simulink model "six_rod_tensegrity_model_2021a"  (R2021a)
settings: Solver=ode45  StartTime=0  StopTime=Inf  RelTol=1e-1
values from neighbouring files (symbols this model uses):
  grivity_z = -9.80665    [code_for_6_rods_tensegrity.m]
  i = 19    [drive_params.m]
  Jsum = Jd + Jp + Jnagr    (= 9.27e-08)    [drive_params.m]
  km = 9.32 / 1000    (= 0.00932)    [drive_params.m]
  kpdr = 0.81    [drive_params.m]
  kw = 60 / (2*pi * 1020)    (= 0.00936205547599)    [drive_params.m]
  L = 0.14 / 1000    (= 0.00014)    [drive_params.m]
  load_mass = 0.5    [code_for_6_rods_tensegrity.m]
  plane_offset = -(rod_length/2 + 0.032 + rod_radius)    [code_for_6_rods_tensegrity.m]
  R = 5.3    [drive_params.m]
  rod_end_drive_offset = spool_active_length    (= 0.015)    [code_for_6_rods_tensegrity.m]
  rod_end_mass = 0.05    [code_for_6_rods_tensegrity.m]
  rod_end_mass_with_drive = 0.2    [code_for_6_rods_tensegrity.m]
  rod_mass = 0.028    [code_for_6_rods_tensegrity.m]
  rod_mass_with_drive = 0.038    [code_for_6_rods_tensegrity.m]
  rod_radius = 0.004    [code_for_6_rods_tensegrity.m]
undefined symbols (not defined in the file or in its folder): Left_end_cap_1_1, Left_end_cap_2_3, Left_end_cap_3_5, Left_end_cap_4_7, Left_end_cap_5_9, Left_end_cap_6_11, Right_end_cap_1_2, Right_end_cap_2_4, Right_end_cap_3_6, Right_end_cap_4_8, Right_end_cap_5_10, Right_end_cap_6_12, Rod_center_1, Rod_center_2, Rod_center_3, Rod_center_4, Rod_center_5, Rod_center_6, sigbuilder_block, X, Y, Z
libraries: sm_lib x403, nesl_utility x73
(part 2 of 5)

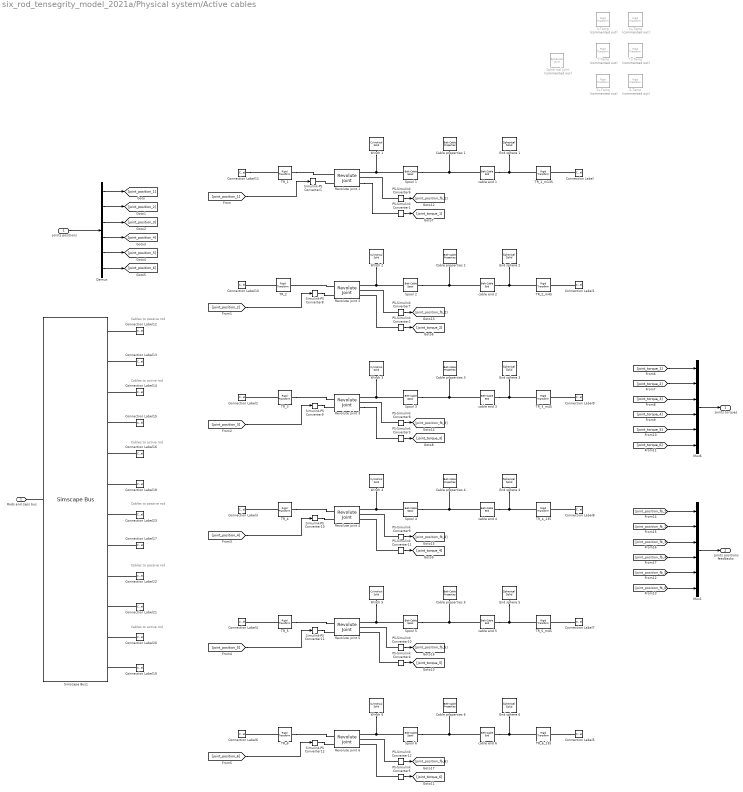
== system six_rod_tensegrity_model_2021a/Physical system/Active cables ==
  note: Cables to passive rod
  note: Cables to active rod
  note: Cables to active rod
  note: Cables to passive rod
  note: Cables to passive rod
  note: Cables to active rod
  Joints positions : Inport
  Cable properties {1..6} (6 alike) : sm_lib/Belts and Cables/Belt-Cable Properties  DrumBeltCableAlignment=Unrestricted  GraphicType=PitchLine  GraphicVisPropType=SimpleVisualProperties  GraphicDiffuseColor=cable_color  GraphicSpecularColor=[0.5 0.5 0.5 1.0]  GraphicAmbientColor=[0.15 0.15 0.15 1.0]  GraphicEmissiveColor=[0.0 0.0 0.0 1.0]  GraphicShininess=75  GraphicOpacity=1
      settings: SourceProductBaseCode=MS
  Connection Label : ConnectionLabel  Label=Cable_left_1_1
  Connection Label1 : ConnectionLabel  Label=Cable_left_2_2
  Connection Label10 : ConnectionLabel  Label=Cable_right_2_6
  Connection Label11 : ConnectionLabel  Label=Cable_right_1_12
  Connection Label12 : ConnectionLabel  Label=Cable_left_1_1
  Connection Label13 : ConnectionLabel  Label=Cable_left_2_2
  Connection Label14 : ConnectionLabel  Label=Cable_left_3_3
  Connection Label15 : ConnectionLabel  Label=Cable_left_4_4
  Connection Label16 : ConnectionLabel  Label=Cable_left_5_5
  Connection Label17 : ConnectionLabel  Label=Cable_left_6_8
  Connection Label18 : ConnectionLabel  Label=Cable_right_2_6
  Connection Label19 : ConnectionLabel  Label=Cable_right_1_12
  Connection Label2 : ConnectionLabel  Label=Cable_left_3_3
  Connection Label20 : ConnectionLabel  Label=Cable_right_6_11
  Connection Label21 : ConnectionLabel  Label=Cable_right_5_10
  Connection Label22 : ConnectionLabel  Label=Cable_right_4_9
  Connection Label23 : ConnectionLabel  Label=Cable_right_3_7
  Connection Label3 : ConnectionLabel  Label=Cable_left_4_4
  Connection Label4 : ConnectionLabel  Label=Cable_left_5_5
  Connection Label5 : ConnectionLabel  Label=Cable_left_6_8
  Connection Label6 : ConnectionLabel  Label=Cable_right_6_11
  Connection Label7 : ConnectionLabel  Label=Cable_right_5_10
  Connection Label8 : ConnectionLabel  Label=Cable_right_4_9
  Connection Label9 : ConnectionLabel  Label=Cable_right_3_7
  Demux : Demux  Outputs=6
  End sphere {1..6} (6 alike) : sm_lib/Body Elements/Spherical Solid  GraphicAmbientColor=[0.15 0.15 0.15 1.0]  BasedOnType=Density  CenterOfMass=[0 0 0]  CenterOfMassUnits=m  GraphicDiffuseColor=spool_color  Density=spool_active_density  DensityUnits=kg/m^3  DoExposeReferenceFrame=on  GraphicEmissiveColor=[0.0 0.0 0.0 1.0]  ExportEntireGeometry=off  SerializedExposedGeometries=<ExposedGeometries/>  SerializedFrames=<Frames/>  MarkerShape=Frame  MarkerSize=10  GraphicType=FromGeometry  InertiaType=CalculateFromGeometry  Mass=0.01  MassUnits=kg  MomentsOfInertia=[1 1 1]  MomentsOfInertiaUnits=kg*m^2  GraphicOpacity=1.0  ProductsOfInertia=[0 0 0]  ProductsOfInertiaUnits=kg*m^2  GraphicShininess=10  GraphicSpecularColor=[0.8 0.8 0.8]  SphereRadius=spool_active_end_radius  SphereRadiusUnits=m  GraphicVisPropType=SimpleVisualProperties
  Mux1 : Mux  Inputs=6
  Mux6 : Mux  Inputs=6
  PS-Simulink Converter{1..5,11} (6 alike) : nesl_utility/PS-Simulink Converter  PhysicalDomain=network_engine_domain  SubClassName=ps_output  LeftPortType=input  RightPortType=output  PseudoPeriodic=off  Frequencies=[]  Unit=N*m  AffineConversion=off
      settings: SourceProductBaseCode=PW,SS
  PS-Simulink Converter{6..10,12} (6 alike) : nesl_utility/PS-Simulink Converter  PhysicalDomain=network_engine_domain  SubClassName=ps_output  LeftPortType=input  RightPortType=output  PseudoPeriodic=off  Frequencies=[]  Unit=rad  AffineConversion=off
      settings: SourceProductBaseCode=PW,SS
  Revolute joint {1..6} (6 alike) : sm_lib/Joints/Revolute Joint  JointMode=Normal  SenseConstraintForce=off  SenseConstraintForceX=off  SenseConstraintForceY=off  SenseConstraintForceZ=off  SenseConstraintTorque=off  SenseConstraintTorqueX=off  SenseConstraintTorqueY=off  SenseConstraintTorqueZ=off  SenseTotalForce=off  SenseTotalForceX=off  SenseTotalForceY=off  SenseTotalForceZ=off  SenseTotalTorque=off  SenseTotalTorqueX=off  SenseTotalTorqueY=off  SenseTotalTorqueZ=off  CompositeWrenchDir=FollowerOnBase  CompositeWrenchFrame=BaseFrame  EquilibriumPosition=0  EquilibriumPositionUnits=deg  SpringStiffness=0  SpringStiffnessUnits=N*m/deg  DampingCoefficient=0  DampingCoefficientUnits=N*m/(deg/s)  TorqueActuationMode=ComputedTorque  MotionActuationMode=InputMotion  SensePosition=on  SenseVelocity=off  SenseAcceleration=off  SenseTorqueForce=on  SenseLowerLimitTorqueForce=off  SenseUpperLimitTorqueForce=off  LowerLimitSpecify=off  LowerLimitBound=-90  LowerLimitBoundUnits=deg  LowerLimitStiffness=1e4  LowerLimitStiffnessUnits=N*m/deg  LowerLimitDamping=10  LowerLimitDampingUnits=N*m/(deg/s)  LowerLimitTransitionRegionWidth=0.1  LowerLimitTransitionRegionWidthUnits=deg  UpperLimitSpecify=off  UpperLimitBound=90  UpperLimitBoundUnits=deg  UpperLimitStiffness=1e4  UpperLimitStiffnessUnits=N*m/deg  UpperLimitDamping=10  UpperLimitDampingUnits=N*m/(deg/s)  UpperLimitTransitionRegionWidth=0.1  UpperLimitTransitionRegionWidthUnits=deg  PositionTargetSpecify=off  PositionTargetPriority=High  PositionTargetValue=0  PositionTargetValueUnits=deg  VelocityTargetSpecify=off  VelocityTargetPriority=High  VelocityTargetValue=0  VelocityTargetValueUnits=deg/s
  Simscape Bus1 : SimscapeBus  HierarchyStrings=Left_end_cap_1_1;Right_end_cap_1_2;Left_end_cap_2_3;Right_end_cap_2_4;Left_end_cap_3_5;Right_end_cap_3_6;Left_end_cap_4_7;Right_end_cap_4_8;Left_end_cap_5_9;Right_end_cap_5_10;Left_end_cap_6_11;Right_end_cap_6_12
  Simulink-PS Converter{1,8..12} (6 alike) : nesl_utility/Simulink-PS Converter  PhysicalDomain=network_engine_domain  SubClassName=ps_input  LeftPortType=input  RightPortType=output  PseudoPeriodic=off  Frequencies=[]  NoiseDistribution=none  NoiseParameters=[]  Unit=rad  AffineConversion=off  FilteringAndDerivatives=filter  SimscapeFilterOrder=2  InputFilterTimeConstant=input_filtering_time  UdotUserProvided=0
      settings: SourceProductBaseCode=PW,SS
  Spherical Joint : sm_lib/Joints/Spherical Joint  Commented=on  JointMode=Normal  SenseConstraintForce=off  SenseConstraintForceX=off  SenseConstraintForceY=off  SenseConstraintForceZ=off  SenseConstraintTorque=off  SenseConstraintTorqueX=off  SenseConstraintTorqueY=off  SenseConstraintTorqueZ=off  SenseTotalForce=off  SenseTotalForceX=off  SenseTotalForceY=off  SenseTotalForceZ=off  SenseTotalTorque=off  SenseTotalTorqueX=off  SenseTotalTorqueY=off  SenseTotalTorqueZ=off  CompositeWrenchDir=FollowerOnBase  CompositeWrenchFrame=BaseFrame  DefPosRotationMethod=None  DefPosRotationAngleUnits=deg  DefPosRotationStandardAxis=+Z  DefPosRotationAngle=0.0  DefPosRotationArbitraryAxis=[0 0 1]  DefPosFollAlignAxisA=+X  DefPosBaseAlignAxisA=+Y  DefPosFollAlignAxisB=+Y  DefPosBaseAlignAxisB=+Z  DefPosRotationSequenceAxes=FollowerAxes  DefPosRotationSequence=XYX  DefPosRotationSequenceAngles=[0 0 0]  DefPosRotationSequenceAnglesUnits=deg  DefPosRotationMatrix=[1 0 0; 0 1 0; 0 0 1]  EqPosRotationMethod=None  EqPosRotationAngleUnits=deg  EqPosRotationStandardAxis=+Z  EqPosRotationAngle=0.0  EqPosRotationArbitraryAxis=[0 0 1]  EqPosFollAlignAxisA=+X  EqPosBaseAlignAxisA=+Y  EqPosFollAlignAxisB=+Y  EqPosBaseAlignAxisB=+Z  EqPosRotationSequenceAxes=FollowerAxes  EqPosRotationSequence=XYX  EqPosRotationSequenceAngles=[0 0 0]  EqPosRotationSequenceAnglesUnits=deg  EqPosRotationMatrix=[1 0 0; 0 1 0; 0 0 1]  SpringStiffness=0  SpringStiffnessUnits=N*m/deg  DampingCoefficient=0  DampingCoefficientUnits=N*m/(deg/s)  ActuateTorqueX=off  ActuateTorqueY=off  ActuateTorqueZ=off  ActuateTorque=off  TorqueActuationMode=NoTorque  MotionActuationMode=ComputedMotion  ActuationFrame=BaseFrame  SensePosition=off  SenseVelocityX=off  SenseVelocityY=off  SenseVelocityZ=off  SenseVelocity=off  SenseAccelerationX=off  SenseAccelerationY=off  SenseAccelerationZ=off  SenseAcceleration=off  SenseTorqueX=off  SenseTorqueY=off  SenseTorqueZ=off  SenseTorqueForce=off  SenseLowerLimitTorqueMag=off  SenseUpperLimitTorqueMag=off  SensingFrame=BaseFrame  LowerLimitSpecify=off  LowerLimitBound=15  LowerLimitBoundUnits=deg  LowerLimitStiffness=1e4  LowerLimitStiffnessUnits=N*m/deg  LowerLimitDamping=10  LowerLimitDampingUnits=N*m/(deg/s)  LowerLimitTransitionRegionWidth=0.1  LowerLimitTransitionRegionWidthUnits=deg  UpperLimitSpecify=off  UpperLimitBound=45  UpperLimitBoundUnits=deg  UpperLimitStiffness=1e4  UpperLimitStiffnessUnits=N*m/deg  UpperLimitDamping=10  UpperLimitDampingUnits=N*m/(deg/s)  UpperLimitTransitionRegionWidth=0.1  UpperLimitTransitionRegionWidthUnits=deg  PositionTargetRotationMethod=None  PositionTargetRotationAngleUnits=deg  PositionTargetRotationStandardAxis=+Z  PositionTargetRotationAngle=0.0  PositionTargetRotationArbitraryAxis=[0 0 1]  PositionTargetFollAlignAxisA=+X  PositionTargetBaseAlignAxisA=+Y  PositionTargetFollAlignAxisB=+Y  PositionTargetBaseAlignAxisB=+Z  PositionTargetRotationSequenceAxes=FollowerAxes  PositionTargetRotationSequence=XYX  PositionTargetRotationSequenceAngles=[0 0 0]  PositionTargetRotationSequenceAnglesUnits=deg  PositionTargetRotationMatrix=[1 0 0; 0 1 0; 0 0 1]  PositionTargetSpecify=off  PositionTargetPriority=High  VelocityTargetValue=[0 0 0]  VelocityTargetValueUnits=deg/s  VelocityTargetSpecify=off  VelocityTargetPriority=High  VelocityTargetInFollowerFrame=on
  Spool {1..6} (6 alike) : sm_lib/Belts and Cables/Belt-Cable Spool  PitchRadius=spool_active_radius  PitchRadiusUnits=m  SenseSpoolAngleA=off  SenseFleetAngleA=off
      settings: SourceProductBaseCode=MS
  TR_1 : sm_lib/Frames and Transforms/Rigid Transform  TranslationMethod=StandardAxis  TranslationStandardOffset=rod_end_drive_offset/2  TranslationLengthUnit=m  TranslationStandardAxis=+Z  TranslationCartesianOffset=[0 0 0]  TranslationROffset=0  TranslationROffsetUnits=m  TranslationZOffset=0  TranslationZOffsetUnits=m  TranslationThetaOffset=0  TranslationThetaOffsetUnits=deg  RotationMethod=None  RotationAngleUnits=deg  RotationStandardAxis=-Y  RotationAngle=180  RotationArbitraryAxis=[0 0 1]  FollAlignAxisA=+X  BaseAlignAxisA=+Y  FollAlignAxisB=+Y  BaseAlignAxisB=+Z  RotationSequenceAxes=FollowerAxes  RotationSequence=XYX  RotationSequenceAngles=[0 0 0]  RotationSequenceAnglesUnits=deg  RotationMatrix=[1 0 0; 0 1 0; 0 0 1]
  TR_1_m135 : sm_lib/Frames and Transforms/Rigid Transform  TranslationMethod=Cylindrical  TranslationStandardOffset=rod_radius  TranslationLengthUnit=m  TranslationStandardAxis=-Z  TranslationCartesianOffset=[rod_radius rod_radius 0]  TranslationROffset=rod_radius  TranslationROffsetUnits=m  TranslationZOffset=0  TranslationZOffsetUnits=m  TranslationThetaOffset=-135  TranslationThetaOffsetUnits=deg  RotationMethod=None  RotationAngleUnits=deg  RotationStandardAxis=+Z  RotationAngle=0.0  RotationArbitraryAxis=[0 0 1]  FollAlignAxisA=+X  BaseAlignAxisA=+Y  FollAlignAxisB=+Y  BaseAlignAxisB=+Z  RotationSequenceAxes=FollowerAxes  RotationSequence=XYX  RotationSequenceAngles=[0 0 0]  RotationSequenceAnglesUnits=deg  RotationMatrix=[1 0 0; 0 1 0; 0 0 1]
  TR_2 : sm_lib/Frames and Transforms/Rigid Transform  TranslationMethod=StandardAxis  TranslationStandardOffset=rod_end_drive_offset/2  TranslationLengthUnit=m  TranslationStandardAxis=+Z  TranslationCartesianOffset=[0 0 0]  TranslationROffset=0  TranslationROffsetUnits=m  TranslationZOffset=0  TranslationZOffsetUnits=m  TranslationThetaOffset=0  TranslationThetaOffsetUnits=deg  RotationMethod=None  RotationAngleUnits=deg  RotationStandardAxis=-Y  RotationAngle=180  RotationArbitraryAxis=[0 0 1]  FollAlignAxisA=+X  BaseAlignAxisA=+Y  FollAlignAxisB=+Y  BaseAlignAxisB=+Z  RotationSequenceAxes=FollowerAxes  RotationSequence=XYX  RotationSequenceAngles=[0 0 0]  RotationSequenceAnglesUnits=deg  RotationMatrix=[1 0 0; 0 1 0; 0 0 1]
  TR_2_m45 : sm_lib/Frames and Transforms/Rigid Transform  TranslationMethod=Cylindrical  TranslationStandardOffset=rod_radius  TranslationLengthUnit=m  TranslationStandardAxis=-Z  TranslationCartesianOffset=[rod_radius rod_radius 0]  TranslationROffset=rod_radius  TranslationROffsetUnits=m  TranslationZOffset=0  TranslationZOffsetUnits=m  TranslationThetaOffset=-45  TranslationThetaOffsetUnits=deg  RotationMethod=None  RotationAngleUnits=deg  RotationStandardAxis=+Z  RotationAngle=0.0  RotationArbitraryAxis=[0 0 1]  FollAlignAxisA=+X  BaseAlignAxisA=+Y  FollAlignAxisB=+Y  BaseAlignAxisB=+Z  RotationSequenceAxes=FollowerAxes  RotationSequence=XYX  RotationSequenceAngles=[0 0 0]  RotationSequenceAnglesUnits=deg  RotationMatrix=[1 0 0; 0 1 0; 0 0 1]
  TR_3 : sm_lib/Frames and Transforms/Rigid Transform  TranslationMethod=StandardAxis  TranslationStandardOffset=rod_end_drive_offset/2  TranslationLengthUnit=m  TranslationStandardAxis=-Z  TranslationCartesianOffset=[0 0 0]  TranslationROffset=0  TranslationROffsetUnits=m  TranslationZOffset=0  TranslationZOffsetUnits=m  TranslationThetaOffset=0  TranslationThetaOffsetUnits=deg  RotationMethod=None  RotationAngleUnits=deg  RotationStandardAxis=-Y  RotationAngle=180  RotationArbitraryAxis=[0 0 1]  FollAlignAxisA=+X  BaseAlignAxisA=+Y  FollAlignAxisB=+Y  BaseAlignAxisB=+Z  RotationSequenceAxes=FollowerAxes  RotationSequence=XYX  RotationSequenceAngles=[0 0 0]  RotationSequenceAnglesUnits=deg  RotationMatrix=[1 0 0; 0 1 0; 0 0 1]
  TR_3_m45 : sm_lib/Frames and Transforms/Rigid Transform  TranslationMethod=Cylindrical  TranslationStandardOffset=rod_radius  TranslationLengthUnit=m  TranslationStandardAxis=-Z  TranslationCartesianOffset=[rod_radius rod_radius 0]  TranslationROffset=rod_radius  TranslationROffsetUnits=m  TranslationZOffset=0  TranslationZOffsetUnits=m  TranslationThetaOffset=-45  TranslationThetaOffsetUnits=deg  RotationMethod=None  RotationAngleUnits=deg  RotationStandardAxis=+Z  RotationAngle=0.0  RotationArbitraryAxis=[0 0 1]  FollAlignAxisA=+X  BaseAlignAxisA=+Y  FollAlignAxisB=+Y  BaseAlignAxisB=+Z  RotationSequenceAxes=FollowerAxes  RotationSequence=XYX  RotationSequenceAngles=[0 0 0]  RotationSequenceAnglesUnits=deg  RotationMatrix=[1 0 0; 0 1 0; 0 0 1]
  TR_4 : sm_lib/Frames and Transforms/Rigid Transform  TranslationMethod=StandardAxis  TranslationStandardOffset=rod_end_drive_offset/2  TranslationLengthUnit=m  TranslationStandardAxis=+Z  TranslationCartesianOffset=[0 0 0]  TranslationROffset=0  TranslationROffsetUnits=m  TranslationZOffset=0  TranslationZOffsetUnits=m  TranslationThetaOffset=0  TranslationThetaOffsetUnits=deg  RotationMethod=None  RotationAngleUnits=deg  RotationStandardAxis=-Y  RotationAngle=180  RotationArbitraryAxis=[0 0 1]  FollAlignAxisA=+X  BaseAlignAxisA=+Y  FollAlignAxisB=+Y  BaseAlignAxisB=+Z  RotationSequenceAxes=FollowerAxes  RotationSequence=XYX  RotationSequenceAngles=[0 0 0]  RotationSequenceAnglesUnits=deg  RotationMatrix=[1 0 0; 0 1 0; 0 0 1]
  TR_4_135 : sm_lib/Frames and Transforms/Rigid Transform  TranslationMethod=Cylindrical  TranslationStandardOffset=rod_radius  TranslationLengthUnit=m  TranslationStandardAxis=-Z  TranslationCartesianOffset=[rod_radius rod_radius 0]  TranslationROffset=rod_radius  TranslationROffsetUnits=m  TranslationZOffset=0  TranslationZOffsetUnits=m  TranslationThetaOffset=135  TranslationThetaOffsetUnits=deg  RotationMethod=None  RotationAngleUnits=deg  RotationStandardAxis=+Z  RotationAngle=0.0  RotationArbitraryAxis=[0 0 1]  FollAlignAxisA=+X  BaseAlignAxisA=+Y  FollAlignAxisB=+Y  BaseAlignAxisB=+Z  RotationSequenceAxes=FollowerAxes  RotationSequence=XYX  RotationSequenceAngles=[0 0 0]  RotationSequenceAnglesUnits=deg  RotationMatrix=[1 0 0; 0 1 0; 0 0 1]
  TR_5 : sm_lib/Frames and Transforms/Rigid Transform  TranslationMethod=StandardAxis  TranslationStandardOffset=rod_end_drive_offset/2  TranslationLengthUnit=m  TranslationStandardAxis=-Z  TranslationCartesianOffset=[0 0 0]  TranslationROffset=0  TranslationROffsetUnits=m  TranslationZOffset=0  TranslationZOffsetUnits=m  TranslationThetaOffset=0  TranslationThetaOffsetUnits=deg  RotationMethod=None  RotationAngleUnits=deg  RotationStandardAxis=-Y  RotationAngle=180  RotationArbitraryAxis=[0 0 1]  FollAlignAxisA=+X  BaseAlignAxisA=+Y  FollAlignAxisB=+Y  BaseAlignAxisB=+Z  RotationSequenceAxes=FollowerAxes  RotationSequence=XYX  RotationSequenceAngles=[0 0 0]  RotationSequenceAnglesUnits=deg  RotationMatrix=[1 0 0; 0 1 0; 0 0 1]
  TR_5_m45 : sm_lib/Frames and Transforms/Rigid Transform  TranslationMethod=Cylindrical  TranslationStandardOffset=rod_radius  TranslationLengthUnit=m  TranslationStandardAxis=-Z  TranslationCartesianOffset=[rod_radius rod_radius 0]  TranslationROffset=rod_radius  TranslationROffsetUnits=m  TranslationZOffset=0  TranslationZOffsetUnits=m  TranslationThetaOffset=-45  TranslationThetaOffsetUnits=deg  RotationMethod=None  RotationAngleUnits=deg  RotationStandardAxis=+Z  RotationAngle=0.0  RotationArbitraryAxis=[0 0 1]  FollAlignAxisA=+X  BaseAlignAxisA=+Y  FollAlignAxisB=+Y  BaseAlignAxisB=+Z  RotationSequenceAxes=FollowerAxes  RotationSequence=XYX  RotationSequenceAngles=[0 0 0]  RotationSequenceAnglesUnits=deg  RotationMatrix=[1 0 0; 0 1 0; 0 0 1]
  TR_6 : sm_lib/Frames and Transforms/Rigid Transform  TranslationMethod=StandardAxis  TranslationStandardOffset=rod_end_drive_offset/2  TranslationLengthUnit=m  TranslationStandardAxis=-Z  TranslationCartesianOffset=[0 0 0]  TranslationROffset=0  TranslationROffsetUnits=m  TranslationZOffset=0  TranslationZOffsetUnits=m  TranslationThetaOffset=0  TranslationThetaOffsetUnits=deg  RotationMethod=None  RotationAngleUnits=deg  RotationStandardAxis=-Y  RotationAngle=180  RotationArbitraryAxis=[0 0 1]  FollAlignAxisA=+X  BaseAlignAxisA=+Y  FollAlignAxisB=+Y  BaseAlignAxisB=+Z  RotationSequenceAxes=FollowerAxes  RotationSequence=XYX  RotationSequenceAngles=[0 0 0]  RotationSequenceAnglesUnits=deg  RotationMatrix=[1 0 0; 0 1 0; 0 0 1]
  TR_6_135 : sm_lib/Frames and Transforms/Rigid Transform  TranslationMethod=Cylindrical  TranslationStandardOffset=rod_radius  TranslationLengthUnit=m  TranslationStandardAxis=-Z  TranslationCartesianOffset=[rod_radius rod_radius 0]  TranslationROffset=rod_radius  TranslationROffsetUnits=m  TranslationZOffset=0  TranslationZOffsetUnits=m  TranslationThetaOffset=135  TranslationThetaOffsetUnits=deg  RotationMethod=None  RotationAngleUnits=deg  RotationStandardAxis=+Z  RotationAngle=0.0  RotationArbitraryAxis=[0 0 1]  FollAlignAxisA=+X  BaseAlignAxisA=+Y  FollAlignAxisB=+Y  BaseAlignAxisB=+Z  RotationSequenceAxes=FollowerAxes  RotationSequence=XYX  RotationSequenceAngles=[0 0 0]  RotationSequenceAnglesUnits=deg  RotationMatrix=[1 0 0; 0 1 0; 0 0 1]
  Winch {1..6} (6 alike) : sm_lib/Body Elements/Cylindrical Solid  GraphicAmbientColor=[0.15 0.15 0.15 1.0]  BasedOnType=Density  CenterOfMass=[0 0 0]  CenterOfMassUnits=m  GraphicDiffuseColor=spool_color  CylinderLength=spool_active_length  CylinderLengthUnits=m  CylinderRadius=spool_active_radius  CylinderRadiusUnits=m  Density=spool_active_density  DensityUnits=kg/m^3  DoExposeReferenceFrame=on  GraphicEmissiveColor=[0.0 0.0 0.0 1.0]  ExportEntireGeometry=off  SerializedFrames=<Frames/>  MarkerShape=Frame  MarkerSize=10  GraphicType=FromGeometry  InertiaType=CalculateFromGeometry  Mass=0.01  MassUnits=kg  MomentsOfInertia=[1 1 1]  MomentsOfInertiaUnits=kg*m^2  GraphicOpacity=1.0  ProductsOfInertia=[0 0 0]  ProductsOfInertiaUnits=kg*m^2  GraphicShininess=10  GraphicSpecularColor=[0.8 0.8 0.8]  GraphicVisPropType=SimpleVisualProperties
  X+Temp : sm_lib/Frames and Transforms/Rigid Transform  Commented=on  TranslationMethod=StandardAxis  TranslationStandardOffset=rod_radius  TranslationLengthUnit=m  TranslationStandardAxis=+X  TranslationCartesianOffset=[0 0 0]  TranslationROffset=0  TranslationROffsetUnits=m  TranslationZOffset=0  TranslationZOffsetUnits=m  TranslationThetaOffset=0  TranslationThetaOffsetUnits=deg  RotationMethod=None  RotationAngleUnits=deg  RotationStandardAxis=+Z  RotationAngle=0.0  RotationArbitraryAxis=[0 0 1]  FollAlignAxisA=+X  BaseAlignAxisA=+Y  FollAlignAxisB=+Y  BaseAlignAxisB=+Z  RotationSequenceAxes=FollowerAxes  RotationSequence=XYX  RotationSequenceAngles=[0 0 0]  RotationSequenceAnglesUnits=deg  RotationMatrix=[1 0 0; 0 1 0; 0 0 1]
  X-Temp : sm_lib/Frames and Transforms/Rigid Transform  Commented=on  TranslationMethod=StandardAxis  TranslationStandardOffset=rod_radius  TranslationLengthUnit=m  TranslationStandardAxis=-X  TranslationCartesianOffset=[0 0 0]  TranslationROffset=0  TranslationROffsetUnits=m  TranslationZOffset=0  TranslationZOffsetUnits=m  TranslationThetaOffset=0  TranslationThetaOffsetUnits=deg  RotationMethod=None  RotationAngleUnits=deg  RotationStandardAxis=+Z  RotationAngle=0.0  RotationArbitraryAxis=[0 0 1]  FollAlignAxisA=+X  BaseAlignAxisA=+Y  FollAlignAxisB=+Y  BaseAlignAxisB=+Z  RotationSequenceAxes=FollowerAxes  RotationSequence=XYX  RotationSequenceAngles=[0 0 0]  RotationSequenceAnglesUnits=deg  RotationMatrix=[1 0 0; 0 1 0; 0 0 1]
  Y+Temp : sm_lib/Frames and Transforms/Rigid Transform  Commented=on  TranslationMethod=StandardAxis  TranslationStandardOffset=rod_radius  TranslationLengthUnit=m  TranslationStandardAxis=+Y  TranslationCartesianOffset=[0 0 0]  TranslationROffset=0  TranslationROffsetUnits=m  TranslationZOffset=0  TranslationZOffsetUnits=m  TranslationThetaOffset=0  TranslationThetaOffsetUnits=deg  RotationMethod=None  RotationAngleUnits=deg  RotationStandardAxis=+Z  RotationAngle=0.0  RotationArbitraryAxis=[0 0 1]  FollAlignAxisA=+X  BaseAlignAxisA=+Y  FollAlignAxisB=+Y  BaseAlignAxisB=+Z  RotationSequenceAxes=FollowerAxes  RotationSequence=XYX  RotationSequenceAngles=[0 0 0]  RotationSequenceAnglesUnits=deg  RotationMatrix=[1 0 0; 0 1 0; 0 0 1]
  Y-Temp : sm_lib/Frames and Transforms/Rigid Transform  Commented=on  TranslationMethod=StandardAxis  TranslationStandardOffset=rod_radius  TranslationLengthUnit=m  TranslationStandardAxis=-Y  TranslationCartesianOffset=[0 0 0]  TranslationROffset=0  TranslationROffsetUnits=m  TranslationZOffset=0  TranslationZOffsetUnits=m  TranslationThetaOffset=0  TranslationThetaOffsetUnits=deg  RotationMethod=None  RotationAngleUnits=deg  RotationStandardAxis=+Z  RotationAngle=0.0  RotationArbitraryAxis=[0 0 1]  FollAlignAxisA=+X  BaseAlignAxisA=+Y  FollAlignAxisB=+Y  BaseAlignAxisB=+Z  RotationSequenceAxes=FollowerAxes  RotationSequence=XYX  RotationSequenceAngles=[0 0 0]  RotationSequenceAnglesUnits=deg  RotationMatrix=[1 0 0; 0 1 0; 0 0 1]
  Z+Temp : sm_lib/Frames and Transforms/Rigid Transform  Commented=on  TranslationMethod=StandardAxis  TranslationStandardOffset=rod_radius  TranslationLengthUnit=m  TranslationStandardAxis=+Z  TranslationCartesianOffset=[0 0 0]  TranslationROffset=0  TranslationROffsetUnits=m  TranslationZOffset=0  TranslationZOffsetUnits=m  TranslationThetaOffset=0  TranslationThetaOffsetUnits=deg  RotationMethod=None  RotationAngleUnits=deg  RotationStandardAxis=+Z  RotationAngle=0.0  RotationArbitraryAxis=[0 0 1]  FollAlignAxisA=+X  BaseAlignAxisA=+Y  FollAlignAxisB=+Y  BaseAlignAxisB=+Z  RotationSequenceAxes=FollowerAxes  RotationSequence=XYX  RotationSequenceAngles=[0 0 0]  RotationSequenceAnglesUnits=deg  RotationMatrix=[1 0 0; 0 1 0; 0 0 1]
  Z-Temp : sm_lib/Frames and Transforms/Rigid Transform  Commented=on  TranslationMethod=StandardAxis  TranslationStandardOffset=rod_radius  TranslationLengthUnit=m  TranslationStandardAxis=-Z  TranslationCartesianOffset=[0 0 0]  TranslationROffset=0  TranslationROffsetUnits=m  TranslationZOffset=0  TranslationZOffsetUnits=m  TranslationThetaOffset=0  TranslationThetaOffsetUnits=deg  RotationMethod=None  RotationAngleUnits=deg  RotationStandardAxis=+Z  RotationAngle=0.0  RotationArbitraryAxis=[0 0 1]  FollAlignAxisA=+X  BaseAlignAxisA=+Y  FollAlignAxisB=+Y  BaseAlignAxisB=+Z  RotationSequenceAxes=FollowerAxes  RotationSequence=XYX  RotationSequenceAngles=[0 0 0]  RotationSequenceAnglesUnits=deg  RotationMatrix=[1 0 0; 0 1 0; 0 0 1]
  cable end {1..6} (6 alike) : sm_lib/Belts and Cables/Belt-Cable End
      settings: SourceProductBaseCode=MS
  Rods end caps bus : PMIOPort  Side=Left
  Joints torques : Outport
  Joints positions feedbacks : Outport  Port=2
  wires:
  [joint_position_2] -> Simulink-PS Converter8/1
  [joint_position_3] -> Simulink-PS Converter9/1
  [joint_position_4] -> Simulink-PS Converter10/1
  [joint_position_5] -> Simulink-PS Converter11/1
  Demux/1 -> [joint_position_1]
  Demux/2 -> [joint_position_2]
  Demux/3 -> [joint_position_3]
  Demux/4 -> [joint_position_4]
  Demux/5 -> [joint_position_5]
  Demux/6 -> [joint_position_6]
  Joints positions/1 -> Demux/1
  PS-Simulink Converter2/1 -> [joint_torque_2]
  PS-Simulink Converter3/1 -> [joint_torque_3]
  PS-Simulink Converter11/1 -> [joint_torque_4]
  PS-Simulink Converter4/1 -> [joint_torque_5]
  PS-Simulink Converter5/1 -> [joint_torque_6]
  [joint_torque_2] -> Mux6/2
  [joint_torque_1] -> Mux6/1
  [joint_torque_3] -> Mux6/3
  Mux6/1 -> Joints torques/1
  [joint_torque_4] -> Mux6/4
  [joint_torque_5] -> Mux6/5
  [joint_torque_6] -> Mux6/6
  PS-Simulink Converter6/1 -> [joint_position_fb_1]
  PS-Simulink Converter7/1 -> [joint_position_fb_2]
  PS-Simulink Converter8/1 -> [joint_position_fb_3]
  PS-Simulink Converter9/1 -> [joint_position_fb_4]
  PS-Simulink Converter10/1 -> [joint_position_fb_5]
  PS-Simulink Converter12/1 -> [joint_position_fb_6]
  [joint_position_fb_4] -> Mux1/4
  [joint_position_fb_5] -> Mux1/5
  Mux1/1 -> Joints positions feedbacks/1
  [joint_position_fb_3] -> Mux1/3
  [joint_position_fb_1] -> Mux1/1
  [joint_position_fb_2] -> Mux1/2
  [joint_position_fb_6] -> Mux1/6
  [joint_position_6] -> Simulink-PS Converter12/1
  [joint_position_1] -> Simulink-PS Converter1/1
  PS-Simulink Converter1/1 -> [joint_torque_1]
  connections:
  Spool 1/LConn1 -- Winch 1/RConn1 -- Revolute joint 1/RConn1
  Spool 1/RConn1 -- cable end 1/RConn1 -- Cable properties 1/LConn1
  TR_1/RConn1 -- Revolute joint 1/LConn1
  End sphere 1/RConn1 -- TR_1_m135/RConn1 -- cable end 1/LConn1
  Connection Label11/LConn1 -- TR_1/LConn1
  Connection Label/LConn1 -- TR_1_m135/LConn1
  Spool 2/LConn1 -- Winch 2/RConn1 -- Revolute joint 2/RConn1
  Spool 2/RConn1 -- cable end 2/RConn1 -- Cable properties 2/LConn1
  End sphere 2/RConn1 -- TR_2_m45/RConn1 -- cable end 2/LConn1
  Simulink-PS Converter8/RConn1 -- Revolute joint 2/LConn2
  Revolute joint 2/LConn1 -- TR_2/RConn1
  Connection Label1/LConn1 -- TR_2_m45/LConn1
  Spool 3/LConn1 -- Winch 3/RConn1 -- Revolute joint 3/RConn1
  Spool 3/RConn1 -- cable end 3/RConn1 -- Cable properties 3/LConn1
  End sphere 3/RConn1 -- TR_3_m45/RConn1 -- cable end 3/LConn1
  Simulink-PS Converter9/RConn1 -- Revolute joint 3/LConn2
  TR_3/LConn1 -- Connection Label2/LConn1
  Connection Label9/LConn1 -- TR_3_m45/LConn1
  TR_3/RConn1 -- Revolute joint 3/LConn1
  Spool 4/LConn1 -- Winch 4/RConn1 -- Revolute joint 4/RConn1
  Spool 4/RConn1 -- cable end 4/RConn1 -- Cable properties 4/LConn1
  End sphere 4/RConn1 -- TR_4_135/RConn1 -- cable end 4/LConn1
  Simulink-PS Converter10/RConn1 -- Revolute joint 4/LConn2
  TR_4/LConn1 -- Connection Label3/LConn1
  Connection Label8/LConn1 -- TR_4_135/LConn1
  TR_4/RConn1 -- Revolute joint 4/LConn1
  Spool 5/LConn1 -- Winch 5/RConn1 -- Revolute joint 5/RConn1
  Spool 5/RConn1 -- cable end 5/RConn1 -- Cable properties 5/LConn1
  End sphere 5/RConn1 -- TR_5_m45/RConn1 -- cable end 5/LConn1
  Simulink-PS Converter11/RConn1 -- Revolute joint 5/LConn2
  TR_5/LConn1 -- Connection Label4/LConn1
  Connection Label7/LConn1 -- TR_5_m45/LConn1
  TR_5/RConn1 -- Revolute joint 5/LConn1
  Spool 6/LConn1 -- Winch 6/RConn1 -- Revolute joint 6/RConn1
  Spool 6/RConn1 -- cable end 6/RConn1 -- Cable properties 6/LConn1
  End sphere 6/RConn1 -- TR_6_135/RConn1 -- cable end 6/LConn1
  Simulink-PS Converter12/RConn1 -- Revolute joint 6/LConn2
  TR_6/LConn1 -- Connection Label6/LConn1
  Connection Label5/LConn1 -- TR_6_135/LConn1
  TR_6/RConn1 -- Revolute joint 6/LConn1
  Connection Label12/LConn1 -- Simscape Bus1/LConn1
  Connection Label13/LConn1 -- Simscape Bus1/LConn2
  Connection Label14/LConn1 -- Simscape Bus1/LConn3
  Connection Label15/LConn1 -- Simscape Bus1/LConn4
  Connection Label16/LConn1 -- Simscape Bus1/LConn5
  Connection Label23/LConn1 -- Simscape Bus1/LConn7
  Connection Label17/LConn1 -- Simscape Bus1/LConn8
  Connection Label22/LConn1 -- Simscape Bus1/LConn9
  Connection Label21/LConn1 -- Simscape Bus1/LConn10
  Connection Label20/LConn1 -- Simscape Bus1/LConn11
  Connection Label19/LConn1 -- Simscape Bus1/LConn12
  Simscape Bus1/RConn1 -- Rods end caps bus/RConn1
  TR_2/LConn1 -- Connection Label10/LConn1
  Connection Label18/LConn1 -- Simscape Bus1/LConn6
  Revolute joint 1/RConn3 -- PS-Simulink Converter1/LConn1
  PS-Simulink Converter6/LConn1 -- Revolute joint 1/RConn2
  PS-Simulink Converter2/LConn1 -- Revolute joint 2/RConn3
  PS-Simulink Converter7/LConn1 -- Revolute joint 2/RConn2
  PS-Simulink Converter8/LConn1 -- Revolute joint 3/RConn2
  Revolute joint 3/RConn3 -- PS-Simulink Converter3/LConn1
  PS-Simulink Converter11/LConn1 -- Revolute joint 4/RConn3
  PS-Simulink Converter9/LConn1 -- Revolute joint 4/RConn2
  PS-Simulink Converter4/LConn1 -- Revolute joint 5/RConn3
  PS-Simulink Converter10/LConn1 -- Revolute joint 5/RConn2
  PS-Simulink Converter5/LConn1 -- Revolute joint 6/RConn3
  PS-Simulink Converter12/LConn1 -- Revolute joint 6/RConn2
  Revolute joint 1/LConn2 -- Simulink-PS Converter1/RConn1

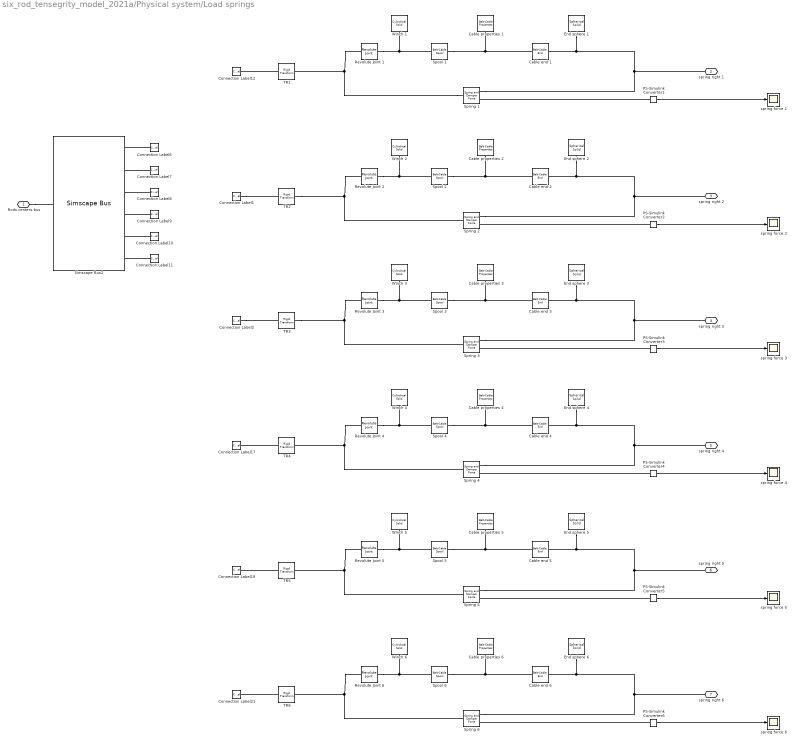
== system six_rod_tensegrity_model_2021a/Physical system/Load springs ==
  Cable properties {1..6} (6 alike) : sm_lib/Belts and Cables/Belt-Cable Properties  DrumBeltCableAlignment=Unrestricted  GraphicType=PitchLine  GraphicVisPropType=SimpleVisualProperties  GraphicDiffuseColor=load_cable_color  GraphicSpecularColor=[0.5 0.5 0.5 1.0]  GraphicAmbientColor=[0.15 0.15 0.15 1.0]  GraphicEmissiveColor=[0.0 0.0 0.0 1.0]  GraphicShininess=75  GraphicOpacity=load_cable_opacity
      settings: SourceProductBaseCode=MS
  Cable end {1..6} (6 alike) : sm_lib/Belts and Cables/Belt-Cable End
      settings: SourceProductBaseCode=MS
  Connection Label1 : ConnectionLabel  Label=Spring_left_2_2
  Connection Label10 : ConnectionLabel  Label=Spring_left_5_5
  Connection Label11 : ConnectionLabel  Label=Spring_left_6_6
  Connection Label12 : ConnectionLabel  Label=Spring_left_1_1
  Connection Label17 : ConnectionLabel  Label=Spring_left_4_4
  Connection Label19 : ConnectionLabel  Label=Spring_left_5_5
  Connection Label2 : ConnectionLabel  Label=Spring_left_3_3
  Connection Label21 : ConnectionLabel  Label=Spring_left_6_6
  Connection Label6 : ConnectionLabel  Label=Spring_left_1_1
  Connection Label7 : ConnectionLabel  Label=Spring_left_2_2
  Connection Label8 : ConnectionLabel  Label=Spring_left_3_3
  Connection Label9 : ConnectionLabel  Label=Spring_left_4_4
  End sphere {1..6} (6 alike) : sm_lib/Body Elements/Spherical Solid  GraphicAmbientColor=[0.15 0.15 0.15 1.0]  BasedOnType=Density  CenterOfMass=[0 0 0]  CenterOfMassUnits=m  GraphicDiffuseColor=load_spool_color  Density=load_spool_density  DensityUnits=kg/m^3  DoExposeReferenceFrame=on  GraphicEmissiveColor=[0.0 0.0 0.0 1.0]  ExportEntireGeometry=off  SerializedExposedGeometries=<ExposedGeometries/>  SerializedFrames=<Frames/>  MarkerShape=Frame  MarkerSize=10  GraphicType=FromGeometry  InertiaType=CalculateFromGeometry  Mass=0.01  MassUnits=kg  MomentsOfInertia=[1 1 1]  MomentsOfInertiaUnits=kg*m^2  GraphicOpacity=load_spool_opacity  ProductsOfInertia=[0 0 0]  ProductsOfInertiaUnits=kg*m^2  GraphicShininess=10  GraphicSpecularColor=[0.8 0.8 0.8]  SphereRadius=load_spool_radius  SphereRadiusUnits=m  GraphicVisPropType=SimpleVisualProperties
  PS-Simulink Converter{1..6} (6 alike) : nesl_utility/PS-Simulink Converter  PhysicalDomain=network_engine_domain  SubClassName=ps_output  LeftPortType=input  RightPortType=output  PseudoPeriodic=off  Frequencies=[]  Unit=N  AffineConversion=off
      settings: SourceProductBaseCode=PW,SS
  Revolute Joint {1..6} (6 alike) : sm_lib/Joints/Revolute Joint  JointMode=Normal  SenseConstraintForce=off  SenseConstraintForceX=off  SenseConstraintForceY=off  SenseConstraintForceZ=off  SenseConstraintTorque=off  SenseConstraintTorqueX=off  SenseConstraintTorqueY=off  SenseConstraintTorqueZ=off  SenseTotalForce=off  SenseTotalForceX=off  SenseTotalForceY=off  SenseTotalForceZ=off  SenseTotalTorque=off  SenseTotalTorqueX=off  SenseTotalTorqueY=off  SenseTotalTorqueZ=off  CompositeWrenchDir=FollowerOnBase  CompositeWrenchFrame=BaseFrame  EquilibriumPosition=0  EquilibriumPositionUnits=deg  SpringStiffness=0  SpringStiffnessUnits=N*m/deg  DampingCoefficient=0  DampingCoefficientUnits=N*m/(deg/s)  TorqueActuationMode=NoTorque  MotionActuationMode=ComputedMotion  SensePosition=off  SenseVelocity=off  SenseAcceleration=off  SenseTorqueForce=off  SenseLowerLimitTorqueForce=off  SenseUpperLimitTorqueForce=off  LowerLimitSpecify=off  LowerLimitBound=-90  LowerLimitBoundUnits=deg  LowerLimitStiffness=1e4  LowerLimitStiffnessUnits=N*m/deg  LowerLimitDamping=10  LowerLimitDampingUnits=N*m/(deg/s)  LowerLimitTransitionRegionWidth=0.1  LowerLimitTransitionRegionWidthUnits=deg  UpperLimitSpecify=off  UpperLimitBound=90  UpperLimitBoundUnits=deg  UpperLimitStiffness=1e4  UpperLimitStiffnessUnits=N*m/deg  UpperLimitDamping=10  UpperLimitDampingUnits=N*m/(deg/s)  UpperLimitTransitionRegionWidth=0.1  UpperLimitTransitionRegionWidthUnits=deg  PositionTargetSpecify=off  PositionTargetPriority=High  PositionTargetValue=0  PositionTargetValueUnits=deg  VelocityTargetSpecify=off  VelocityTargetPriority=High  VelocityTargetValue=0  VelocityTargetValueUnits=deg/s
  Simscape Bus2 : SimscapeBus  HierarchyStrings=Rod_center_1;Rod_center_2;Rod_center_3;Rod_center_4;Rod_center_5;Rod_center_6
  Spool {1..6} (6 alike) : sm_lib/Belts and Cables/Belt-Cable Spool  PitchRadius=load_spool_radius  PitchRadiusUnits=m  SenseSpoolAngleA=off  SenseFleetAngleA=off
      settings: SourceProductBaseCode=MS
  Spring 1 : sm_lib/Forces and Torques/Spring and Damper Force  NaturalLength=load_spring_natural_length_1  NaturalLengthUnits=m  SpringStiffness=load_spring_stiffness  SpringStiffnessUnits=N/m  DampingCoefficient=load_spring_damping  DampingCoefficientUnits=N/(m/s)  SenseForce=on
  Spring 2 : sm_lib/Forces and Torques/Spring and Damper Force  NaturalLength=load_spring_natural_length_2  NaturalLengthUnits=m  SpringStiffness=load_spring_stiffness  SpringStiffnessUnits=N/m  DampingCoefficient=load_spring_damping  DampingCoefficientUnits=N/(m/s)  SenseForce=on
  Spring 3 : sm_lib/Forces and Torques/Spring and Damper Force  NaturalLength=load_spring_natural_length_3  NaturalLengthUnits=m  SpringStiffness=load_spring_stiffness  SpringStiffnessUnits=N/m  DampingCoefficient=load_spring_damping  DampingCoefficientUnits=N/(m/s)  SenseForce=on
  Spring 4 : sm_lib/Forces and Torques/Spring and Damper Force  NaturalLength=load_spring_natural_length_4  NaturalLengthUnits=m  SpringStiffness=load_spring_stiffness  SpringStiffnessUnits=N/m  DampingCoefficient=load_spring_damping  DampingCoefficientUnits=N/(m/s)  SenseForce=on
  Spring 5 : sm_lib/Forces and Torques/Spring and Damper Force  NaturalLength=load_spring_natural_length_5  NaturalLengthUnits=m  SpringStiffness=load_spring_stiffness  SpringStiffnessUnits=N/m  DampingCoefficient=load_spring_damping  DampingCoefficientUnits=N/(m/s)  SenseForce=on
  Spring 6 : sm_lib/Forces and Torques/Spring and Damper Force  NaturalLength=load_spring_natural_length_6  NaturalLengthUnits=m  SpringStiffness=load_spring_stiffness  SpringStiffnessUnits=N/m  DampingCoefficient=load_spring_damping  DampingCoefficientUnits=N/(m/s)  SenseForce=on
  TR1 : sm_lib/Frames and Transforms/Rigid Transform  TranslationMethod=StandardAxis  TranslationStandardOffset=rod_radius  TranslationLengthUnit=m  TranslationStandardAxis=+X  TranslationCartesianOffset=[0 0 0]  TranslationROffset=0  TranslationROffsetUnits=m  TranslationZOffset=0  TranslationZOffsetUnits=m  TranslationThetaOffset=0  TranslationThetaOffsetUnits=deg  RotationMethod=None  RotationAngleUnits=deg  RotationStandardAxis=-Y  RotationAngle=90  RotationArbitraryAxis=[0 0 1]  FollAlignAxisA=+X  BaseAlignAxisA=+Y  FollAlignAxisB=+Y  BaseAlignAxisB=+Z  RotationSequenceAxes=FollowerAxes  RotationSequence=XYX  RotationSequenceAngles=[0 0 0]  RotationSequenceAnglesUnits=deg  RotationMatrix=[1 0 0; 0 1 0; 0 0 1]
  TR2 : sm_lib/Frames and Transforms/Rigid Transform  TranslationMethod=StandardAxis  TranslationStandardOffset=rod_radius  TranslationLengthUnit=m  TranslationStandardAxis=-X  TranslationCartesianOffset=[0 0 0]  TranslationROffset=0  TranslationROffsetUnits=m  TranslationZOffset=0  TranslationZOffsetUnits=m  TranslationThetaOffset=0  TranslationThetaOffsetUnits=deg  RotationMethod=None  RotationAngleUnits=deg  RotationStandardAxis=-Y  RotationAngle=90  RotationArbitraryAxis=[0 0 1]  FollAlignAxisA=+X  BaseAlignAxisA=+Y  FollAlignAxisB=+Y  BaseAlignAxisB=+Z  RotationSequenceAxes=FollowerAxes  RotationSequence=XYX  RotationSequenceAngles=[0 0 0]  RotationSequenceAnglesUnits=deg  RotationMatrix=[1 0 0; 0 1 0; 0 0 1]
  TR3 : sm_lib/Frames and Transforms/Rigid Transform  TranslationMethod=StandardAxis  TranslationStandardOffset=rod_radius  TranslationLengthUnit=m  TranslationStandardAxis=+Y  TranslationCartesianOffset=[0 0 0]  TranslationROffset=0  TranslationROffsetUnits=m  TranslationZOffset=0  TranslationZOffsetUnits=m  TranslationThetaOffset=0  TranslationThetaOffsetUnits=deg  RotationMethod=None  RotationAngleUnits=deg  RotationStandardAxis=-Y  RotationAngle=90  RotationArbitraryAxis=[0 0 1]  FollAlignAxisA=+X  BaseAlignAxisA=+Y  FollAlignAxisB=+Y  BaseAlignAxisB=+Z  RotationSequenceAxes=FollowerAxes  RotationSequence=XYX  RotationSequenceAngles=[0 0 0]  RotationSequenceAnglesUnits=deg  RotationMatrix=[1 0 0; 0 1 0; 0 0 1]
  TR4 : sm_lib/Frames and Transforms/Rigid Transform  TranslationMethod=StandardAxis  TranslationStandardOffset=rod_radius  TranslationLengthUnit=m  TranslationStandardAxis=-Y  TranslationCartesianOffset=[0 0 0]  TranslationROffset=0  TranslationROffsetUnits=m  TranslationZOffset=0  TranslationZOffsetUnits=m  TranslationThetaOffset=0  TranslationThetaOffsetUnits=deg  RotationMethod=None  RotationAngleUnits=deg  RotationStandardAxis=-Y  RotationAngle=90  RotationArbitraryAxis=[0 0 1]  FollAlignAxisA=+X  BaseAlignAxisA=+Y  FollAlignAxisB=+Y  BaseAlignAxisB=+Z  RotationSequenceAxes=FollowerAxes  RotationSequence=XYX  RotationSequenceAngles=[0 0 0]  RotationSequenceAnglesUnits=deg  RotationMatrix=[1 0 0; 0 1 0; 0 0 1]
  TR5 : sm_lib/Frames and Transforms/Rigid Transform  TranslationMethod=StandardAxis  TranslationStandardOffset=rod_radius  TranslationLengthUnit=m  TranslationStandardAxis=+X  TranslationCartesianOffset=[0 0 0]  TranslationROffset=0  TranslationROffsetUnits=m  TranslationZOffset=0  TranslationZOffsetUnits=m  TranslationThetaOffset=0  TranslationThetaOffsetUnits=deg  RotationMethod=None  RotationAngleUnits=deg  RotationStandardAxis=-Y  RotationAngle=90  RotationArbitraryAxis=[0 0 1]  FollAlignAxisA=+X  BaseAlignAxisA=+Y  FollAlignAxisB=+Y  BaseAlignAxisB=+Z  RotationSequenceAxes=FollowerAxes  RotationSequence=XYX  RotationSequenceAngles=[0 0 0]  RotationSequenceAnglesUnits=deg  RotationMatrix=[1 0 0; 0 1 0; 0 0 1]
  TR6 : sm_lib/Frames and Transforms/Rigid Transform  TranslationMethod=StandardAxis  TranslationStandardOffset=rod_radius  TranslationLengthUnit=m  TranslationStandardAxis=-X  TranslationCartesianOffset=[0 0 0]  TranslationROffset=0  TranslationROffsetUnits=m  TranslationZOffset=0  TranslationZOffsetUnits=m  TranslationThetaOffset=0  TranslationThetaOffsetUnits=deg  RotationMethod=None  RotationAngleUnits=deg  RotationStandardAxis=-Y  RotationAngle=90  RotationArbitraryAxis=[0 0 1]  FollAlignAxisA=+X  BaseAlignAxisA=+Y  FollAlignAxisB=+Y  BaseAlignAxisB=+Z  RotationSequenceAxes=FollowerAxes  RotationSequence=XYX  RotationSequenceAngles=[0 0 0]  RotationSequenceAnglesUnits=deg  RotationMatrix=[1 0 0; 0 1 0; 0 0 1]
  Winch {1..6} (6 alike) : sm_lib/Body Elements/Cylindrical Solid  GraphicAmbientColor=[0.15 0.15 0.15 1.0]  BasedOnType=Density  CenterOfMass=[0 0 0]  CenterOfMassUnits=m  GraphicDiffuseColor=load_spool_color  CylinderLength=load_spool_length  CylinderLengthUnits=m  CylinderRadius=load_spool_radius  CylinderRadiusUnits=m  Density=load_spool_density  DensityUnits=kg/m^3  DoExposeReferenceFrame=on  GraphicEmissiveColor=[0.0 0.0 0.0 1.0]  ExportEntireGeometry=off  SerializedFrames=<Frames/>  MarkerShape=Frame  MarkerSize=10  GraphicType=FromGeometry  InertiaType=CalculateFromGeometry  Mass=0.01  MassUnits=kg  MomentsOfInertia=[1 1 1]  MomentsOfInertiaUnits=kg*m^2  GraphicOpacity=load_spool_opacity  ProductsOfInertia=[0 0 0]  ProductsOfInertiaUnits=kg*m^2  GraphicShininess=10  GraphicSpecularColor=[0.8 0.8 0.8]  GraphicVisPropType=SimpleVisualProperties
  spring force {1..6} (6 alike) : Scope
  Rods centers bus : PMIOPort  Side=Left
  spring right 1 : PMIOPort  Port=2  Side=Right
  spring right 2 : PMIOPort  Port=3  Side=Right
  spring right 3 : PMIOPort  Port=4  Side=Right
  spring right 4 : PMIOPort  Port=5  Side=Right
  spring right 5 : PMIOPort  Port=6  Side=Right
  spring right 6 : PMIOPort  Port=7  Side=Right
  wires:
  PS-Simulink Converter1/1 -> spring force 1/1
  PS-Simulink Converter2/1 -> spring force 2/1
  PS-Simulink Converter3/1 -> spring force 3/1
  PS-Simulink Converter4/1 -> spring force 4/1
  PS-Simulink Converter5/1 -> spring force 5/1
  PS-Simulink Converter6/1 -> spring force 6/1
  connections:
  Rods centers bus/RConn1 -- Simscape Bus2/RConn1
  Connection Label6/LConn1 -- Simscape Bus2/LConn1
  Connection Label7/LConn1 -- Simscape Bus2/LConn2
  Connection Label8/LConn1 -- Simscape Bus2/LConn3
  Connection Label9/LConn1 -- Simscape Bus2/LConn4
  Connection Label10/LConn1 -- Simscape Bus2/LConn5
  Connection Label11/LConn1 -- Simscape Bus2/LConn6
  Winch 1/RConn1 -- Spool 1/LConn1 -- Revolute Joint 1/RConn1
  Cable properties 1/LConn1 -- Spool 1/RConn1 -- Cable end 1/RConn1
  Spring 1/LConn1 -- Revolute Joint 1/LConn1 -- TR1/RConn1
  Cable end 1/LConn1 -- End sphere 1/RConn1 -- spring right 1/RConn1 -- Spring 1/RConn1
  PS-Simulink Converter1/LConn1 -- Spring 1/RConn2
  Spool 2/LConn1 -- Winch 2/RConn1 -- Revolute Joint 2/RConn1
  Spool 2/RConn1 -- Cable properties 2/LConn1 -- Cable end 2/RConn1
  Connection Label1/LConn1 -- TR2/LConn1
  End sphere 2/RConn1 -- Cable end 2/LConn1 -- spring right 2/RConn1 -- Spring 2/RConn1
  PS-Simulink Converter2/LConn1 -- Spring 2/RConn2
  Winch 3/RConn1 -- Spool 3/LConn1 -- Revolute Joint 3/RConn1
  Cable properties 3/LConn1 -- Spool 3/RConn1 -- Cable end 3/RConn1
  Connection Label2/LConn1 -- TR3/LConn1
  Spring 3/RConn1 -- spring right 3/RConn1 -- End sphere 3/RConn1 -- Cable end 3/LConn1
  PS-Simulink Converter3/LConn1 -- Spring 3/RConn2
  Spool 4/LConn1 -- Winch 4/RConn1 -- Revolute Joint 4/RConn1
  Spool 4/RConn1 -- Cable properties 4/LConn1 -- Cable end 4/RConn1
  Revolute Joint 4/LConn1 -- Spring 4/LConn1 -- TR4/RConn1
  End sphere 4/RConn1 -- spring right 4/RConn1 -- Spring 4/RConn1 -- Cable end 4/LConn1
  PS-Simulink Converter4/LConn1 -- Spring 4/RConn2
  Winch 5/RConn1 -- Spool 5/LConn1 -- Revolute Joint 5/RConn1
  Cable properties 5/LConn1 -- Spool 5/RConn1 -- Cable end 5/RConn1
  TR5/LConn1 -- Connection Label19/LConn1
  Spring 5/RConn1 -- spring right 5/RConn1 -- End sphere 5/RConn1 -- Cable end 5/LConn1
  PS-Simulink Converter5/LConn1 -- Spring 5/RConn2
  Spool 6/LConn1 -- Winch 6/RConn1 -- Revolute Joint 6/RConn1
  Spool 6/RConn1 -- Cable properties 6/LConn1 -- Cable end 6/RConn1
  Revolute Joint 6/LConn1 -- Spring 6/LConn1 -- TR6/RConn1
  End sphere 6/RConn1 -- spring right 6/RConn1 -- Spring 6/RConn1 -- Cable end 6/LConn1
  PS-Simulink Converter6/LConn1 -- Spring 6/RConn2
  TR1/LConn1 -- Connection Label12/LConn1
  Revolute Joint 2/LConn1 -- TR2/RConn1 -- Spring 2/LConn1
  TR3/RConn1 -- Revolute Joint 3/LConn1 -- Spring 3/LConn1
  TR4/LConn1 -- Connection Label17/LConn1
  Revolute Joint 5/LConn1 -- TR5/RConn1 -- Spring 5/LConn1
  TR6/LConn1 -- Connection Label21/LConn1
